simulink model "BLUEFINSHIPDYNAMICS_GEORGEWILL"  (R2018a)
settings: Solver=ode4  StartTime=0.0  StopTime=100  FixedStep=0.001  RelTol=1e-3
InitFcn:
  | u = 0.00399;
  | v= 0;
  | r= 0;
  | psi= 0;
  | del= 0;
  | x= 0;
  | y= 0;
settings Model: Creator=gco0  LastModifiedBy=gco0

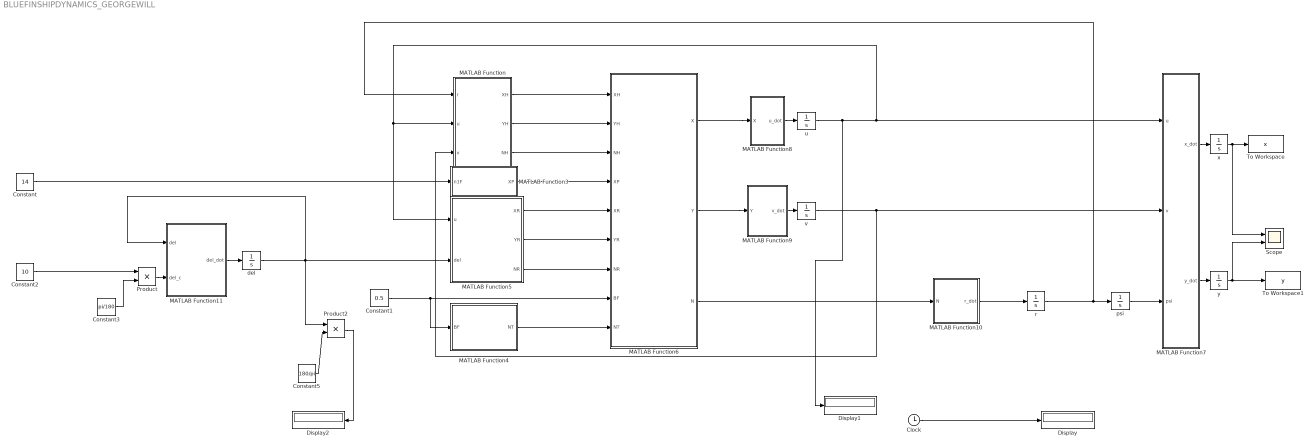
== system BLUEFINSHIPDYNAMICS_GEORGEWILL ==
  Clock : Clock
  Constant : Constant  Value=14  SampleTime=10
  Constant1 : Constant  Value=0.5
  Constant2 : Constant  Value=10
  Constant3 : Constant  Value=pi/180
  Constant5 : Constant  Value=180/pi
  Display : Display
  Display1 : Display
  Display2 : Display
  MATLAB Function : MATLAB Function  TreatAsAtomicUnit=on
  MATLAB Function10 : MATLAB Function  TreatAsAtomicUnit=on
  MATLAB Function11 : MATLAB Function  TreatAsAtomicUnit=on
  MATLAB Function3 : MATLAB Function  TreatAsAtomicUnit=on
  MATLAB Function4 : MATLAB Function  TreatAsAtomicUnit=on
  MATLAB Function5 : MATLAB Function  TreatAsAtomicUnit=on
  MATLAB Function6 : MATLAB Function  TreatAsAtomicUnit=on
  MATLAB Function7 : MATLAB Function  TreatAsAtomicUnit=on
  MATLAB Function8 : MATLAB Function  TreatAsAtomicUnit=on
  MATLAB Function9 : MATLAB Function  TreatAsAtomicUnit=on
  Product : Product
  Product2 : Product
  Scope : Scope  NumInputPorts=2
  To Workspace : ToWorkspace  VariableName=x  SampleTime=-1
  To Workspace1 : ToWorkspace  VariableName=y  SampleTime=-1
  del : Integrator  LimitOutput=on  UpperSaturationLimit=35*pi/180  LowerSaturationLimit=0
  psi : Integrator  UpperSaturationLimit=1  LowerSaturationLimit=0
  r : Integrator  UpperSaturationLimit=35*pi/180  LowerSaturationLimit=-35
  u : Integrator  UpperSaturationLimit=11  LowerSaturationLimit=0
  v : Integrator  UpperSaturationLimit=11  LowerSaturationLimit=0
  x : Integrator  UpperSaturationLimit=35*pi/180  LowerSaturationLimit=-35
  y : Integrator  UpperSaturationLimit=35*pi/180  LowerSaturationLimit=-35
  wires:
  Constant/1 -> MATLAB Function3/1(n1F)
  Constant1/1 -> MATLAB Function4/1(BF), MATLAB Function6/8(BF)
  MATLAB Function/1(XH) -> MATLAB Function6/1(XH)
  MATLAB Function3/1(XP) -> MATLAB Function6/4(XP)
  MATLAB Function5/1(XR) -> MATLAB Function6/5(XR)
  MATLAB Function5/2(YR) -> MATLAB Function6/6(YR)
  MATLAB Function5/3(NR) -> MATLAB Function6/7(NR)
  MATLAB Function4/1(NT) -> MATLAB Function6/9(NT)
  MATLAB Function7/1(x_dot) -> x/1
  Constant2/1 -> Product/1
  Constant3/1 -> Product/2
  MATLAB Function6/1(X) -> MATLAB Function8/1(X)
  MATLAB Function6/2(Y) -> MATLAB Function9/1(Y)
  MATLAB Function6/3(N) -> MATLAB Function10/1(N)
  MATLAB Function10/1(r_dot) -> r/1
  MATLAB Function9/1(v_dot) -> v/1
  MATLAB Function8/1(u_dot) -> u/1
  Product/1 -> MATLAB Function11/2(del_c)
  MATLAB Function11/1(del_dot) -> del/1
  MATLAB Function7/2(y_dot) -> y/1
  v/1 -> MATLAB Function/3(v), MATLAB Function7/2(v)
  MATLAB Function/2(YH) -> MATLAB Function6/2(YH)
  MATLAB Function/3(NH) -> MATLAB Function6/3(NH)
  r/1 -> MATLAB Function/1(r), psi/1
  u/1 -> Display1/1, MATLAB Function5/1(u), MATLAB Function/2(u), MATLAB Function7/1(u)
  Constant5/1 -> Product2/2
  del/1 -> MATLAB Function11/1(del), Product2/1, MATLAB Function5/2(del)
  Product2/1 -> Display2/1
  psi/1 -> MATLAB Function7/3(psi)
  Clock/1 -> Display/1
  x/1 -> To Workspace/1, Scope/1
  y/1 -> To Workspace1/1, Scope/2

== matlab function BLUEFINSHIPDYNAMICS_GEORGEWILL/MATLAB Function ==
  data: r input; u input; XH output; v input; YH output; NH output
function [XH,YH,NH] = HULL(r,u,v)
% System parameters:
% Physical constants:
    rho = 1046.1;       % divided by g = 9.81 m/s^2?
    rhoA= 0.1250;       % divided by g = 9.81 m/s^2?
    g   = 9.81;
    del_max  = 40*pi/180;
    deld_max = 5*pi/180;
    rad = asin(1.0)/90.0;
% Ship
    m  = 64.55;
   % m = m*2/(rho*L*L*L);
    mx = 2.557374;
    my = 5.173345;
    Iz = 10.17;
    
     %Iz = Iz*2/(rho*L*L*L*L*L);
    L  = 1.569;
   %L = L/L;
    d  =  0.193;
    %d = d/d;
    Sw = 480.00;
%  Hull parameters:
    ct = 4.32750e-3;
     Xv = 0.9610;      Yv = 0;        Nv = -0.0000; % by 10 zigzag data
    Xvv = -1.1143;     Yvv = 0.0068;       Nvv = 0.0030;
     Xr = -0.0005;       Yr = -0.0000;        Nr = -0.0000;
     Xrr = -0.0000;      Yrr = -0.0000;       Nrr = -0.0000;
    Xvr = -0.00021;      Yvr = -0.0000;       Nvr = -0.0000;
    
   %  Xv = -0.0278;      Yv = -0.0049;        Nv = 5.2042*(10^-17);
   % Xvv = 0.0133;     Yvv = 0.0095;       Nvv = 0.0030;
   % Xr = -0.0005;       Yr = -0.0001;        Nr = -2.7529*(10^-21);
   % Xrr = -0.0000;      Yrr = -0.0000;       Nrr = -1.4863*(10^-25);
   % Xvr = -0.0000;      Yvr = -0.0000;       Nvr = 7.6233*(10^-21);
 
% Non-dimentional states:
%U = sqrt(u*u+v*v);
U = sqrt(0.06369^2+0.00493^2);   
   
vd = v/U;
rd = r*L/U;


XH =m*v*r-0.5*rho*Sw*ct*abs(u)*u+0.5*rho*L*d*U^2*(Xv*abs(vd)+...
     Xvr*vd*rd+Xv*abs(rd)+Xvv*vd*vd+Xrr*rd*rd);
YH= -m*u+0.5*rho*L*d*(U^2)*(Yv*vd+Yvr*vd*rd+Yr*rd+...
     Yvv*abs(vd)*vd+Yrr*rd*abs(rd));

NH = 0.5*rho*L^2*d*U^2*(Nv*vd+Nvr*abs(vd)*rd+Nr*rd+Nvv*vd*abs(vd)...
     +Nrr*rd*abs(rd));

== matlab function BLUEFINSHIPDYNAMICS_GEORGEWILL/MATLAB Function3 ==
  data: n1F input; XP output
function XP = PROPELLER(n1F)

% Propeller parameters:
    tp = 0.193;
    wp = 0.28989;
    Dp = 2.2;
    Fp = 8.1928;
% Propeller:
%Jp = (1-wp)/(n1*Dp)*u;
%XP = (1-tp)*rho*n1^2*Dp^4;
XP = Fp*2*n1F;
YP = 0;
NP = 0;

== matlab function BLUEFINSHIPDYNAMICS_GEORGEWILL/MATLAB Function4 ==
  data: BF input; NT output
function NT = Thruster(BF)

% Thruster
   % Thb = 0.65e3;
   %Tlb =-18.8;
   %Ft = 10;
   Ft = 1.20834;
   Tlb = 0.38;
% Thrusters:
XT = 0;
%YT = Thb*BT/10;
YT = Ft*4*BF;
NT = Tlb*YT;
%YT = 1.20834;
%NT = 1.20834*0.38;

== matlab function BLUEFINSHIPDYNAMICS_GEORGEWILL/MATLAB Function5 ==
  data: XR output; YR output; u input; NR output; del input
function [XR,YR,NR] = Rudder(u,del)

% Rudder:
%UR = (eps-kx)*(1-wp)*u+kx*0.7*pi*Dp*n1;
%URd = UR/U;
%alR = del+atan(gamR*(vd+lR*rd)/URd);
%FN = 0.5*rho*AR*falp*UR^2*sin(alR);
%FN = 0.5*rho*AR*falp*UR*(UR*sin(del)+(v+lR*L*r)*gamR*cos(del));
%XR = -(1-tr)*FN*sin(del);
%YR = -(1+aH)*FN*cos(del);
%NR = -(xR+aH*xH)*FN*cos(del);

%FN = 576.2*0.475*(u^2);
FN = 576.2*0.0612*(u^2);
XR = FN*sin(del);
YR = FN*cos(del);
NR = 0.7*FN*cos(del);

== matlab function BLUEFINSHIPDYNAMICS_GEORGEWILL/MATLAB Function6 ==
  data: XH input; X output; YH input; NH input; XP input; XR input; YR input; NR input; BF input; NT input; Y output; N output
function [X,Y,N] = forcesmoments(XH,YH,NH,XP,XR,YR,NR,BF,NT)


% Thrututer
Ft = 1.20834;
   
%YT = Thb*BT/10;
YT = Ft*4*BF;


% Thrusters:
XT = 0;

% Propeller:
YP = 0;
NP = 0;

% Forces and moments:
X = XH + XP + XR + XT;
Y = YH + YP + YR + YT;
N = NH + NP + NR + NT;

== matlab function BLUEFINSHIPDYNAMICS_GEORGEWILL/MATLAB Function7 ==
  data: u input; v input; x_dot output; y_dot output; psi input
function [x_dot,y_dot] = trajectory(u,v,psi)

% System parameters:
% Physical constants:
    rho = 1046.1;       % divided by g = 9.81 m/s^2?
    rhoA= 0.1250;       % divided by g = 9.81 m/s^2?
    g   = 9.81;
    del_max  = 40*pi/180;
    deld_max = 5*pi/180;
    rad = asin(1.0)/90.0;
% Ship
    m  = 64.55;
   % m = m*2/(rho*L*L*L);
    mx = 2.557374;
    my = 5.173345;
    Iz = 10.17;
   %Iz = Iz*2/(rho*L*L*L*L*L);
    L  = 1.569;
   %L = L/L;
  


% Rudder parameters:
    Td  = 11.9;
    a  = 1;
 
    
% Masses and moments of inertia:
    %m11 = (m+mx);
   % m22 = (m+my);
    %m33 = Iz; 
    
    m11 = (m+mx);
    m22 = (m+my);
    m33 = Iz;
    
% Non-dimentional states:
%U = sqrt(u*u+v*v);
U = sqrt(0.06369^2+0.00493^2);

x_dot=(u*cos(psi)-v*sin(psi))/U;
y_dot=(u*sin(psi)+v*cos(psi))/U;

== matlab function BLUEFINSHIPDYNAMICS_GEORGEWILL/MATLAB Function8 ==
  data: X input; u_dot output
function u_dot  = surge(X)

% System parameters:
% Physical constants:
    rho = 1046.1;       % divided by g = 9.81 m/s^2?
    rhoA= 0.1250;       % divided by g = 9.81 m/s^2?
    g   = 9.81;
    del_max  = 40*pi/180;
    deld_max = 5*pi/180;
    rad = asin(1.0)/90.0;
% Ship
    m  = 64.55;
   % m = m*2/(rho*L*L*L);
    mx = 2.557374;
    my = 5.173345;
    Iz = 10.17;
   %Iz = Iz*2/(rho*L*L*L*L*L);
    L  = 1.569;
   %L = L/L;
  



 
    
% Masses and moments of inertia:
    %m11 = (m+mx);
   % m22 = (m+my);
    %m33 = Iz; 
    
    m11 = (m+mx);
    m22 = (m+my);
    m33 = Iz;
    % Non-dimentional states:
%U = sqrt(u*u+v*v);
U = sqrt(0.06369^2+0.00493^2);
    
u_dot=X*2/(m11*(rho*L*L*U*U));

== matlab function BLUEFINSHIPDYNAMICS_GEORGEWILL/MATLAB Function9 ==
  data: Y input; v_dot output
function v_dot  = sway(Y)

% System parameters:
% Physical constants:
    rho = 1046.1;       % divided by g = 9.81 m/s^2?
    rhoA= 0.1250;       % divided by g = 9.81 m/s^2?
    g   = 9.81;
    del_max  = 40*pi/180;
    deld_max = 5*pi/180;
    rad = asin(1.0)/90.0;
% Ship
    m  = 64.55;
   % m = m*2/(rho*L*L*L);
    mx = 2.557374;
    my = 5.173345;
    Iz = 10.17;
   %Iz = Iz*2/(rho*L*L*L*L*L);
    L  = 1.569;
   %L = L/L;
  



 
    
% Masses and moments of inertia:
    %m11 = (m+mx);
   % m22 = (m+my);
    %m33 = Iz; 
    
    m11 = (m+mx);
    m22 = (m+my);
    m33 = Iz;
    
% Non-dimentional states:
%U = sqrt(u*u+v*v);
U = sqrt(0.06369^2+0.00493^2);






v_dot=Y*2/(m22*(rho*L*L*U*U));

== matlab function BLUEFINSHIPDYNAMICS_GEORGEWILL/MATLAB Function10 ==
  data: N input; r_dot output
function r_dot  = yawrate(N)

% System parameters:
% Physical constants:
    rho = 1046.1;       % divided by g = 9.81 m/s^2?
    rhoA= 0.1250;       % divided by g = 9.81 m/s^2?
    g   = 9.81;
   
% Ship
    m  = 64.55;
   % m = m*2/(rho*L*L*L);
    mx = 2.557374;
    my = 5.173345;
    Iz = 10.17;
   %Iz = Iz*2/(rho*L*L*L*L*L);
    L  = 1.569;
   %L = L/L;
  



 
    
% Masses and moments of inertia:
    %m11 = (m+mx);
   % m22 = (m+my);
    %m33 = Iz; 
    
    m11 = (m+mx);
    m22 = (m+my);
    m33 = Iz;
    
% Non-dimentional states:
%U = sqrt(u*u+v*v);
U = sqrt(0.06369^2+0.00493^2);






r_dot=N*2/(m33*(rho*L*L*L*U*U));

== matlab function BLUEFINSHIPDYNAMICS_GEORGEWILL/MATLAB Function11 ==
  data: del input; del_dot output; del_c input
function del_dot  = autopilot(del,del_c)

% Rudder parameters:
    Td  = 11.9;
    a  = 1;


del_dot=(del_c-del)/(abs(del_c-del)*Td+a);
